simulink model "StoneVsAir"  (Simulink 7.6)
settings: Solver=ode5  StartTime=0.0  StopTime=10.0  FixedStep=0.01  RelTol=1e-3
libraries: simulink x1
settings Model: Creator=Podolsky  LastModifiedBy=Podolsky
settings DataIOCC: SignalLoggingName=sigsOut
settings DebuggingCC: SaveWithParameterizedLinksMsg=none  SignalResolutionControl=TryResolveAllWithWarning  SolverPrmCheckMsg=none  MultiTaskDSMMsg=warning  MultiTaskCondExecSysMsg=none  StrictBusMsg=None
settings HardwareCC: TargetUnknown=on
settings RTWCC: IncludeERTFirstTime=on

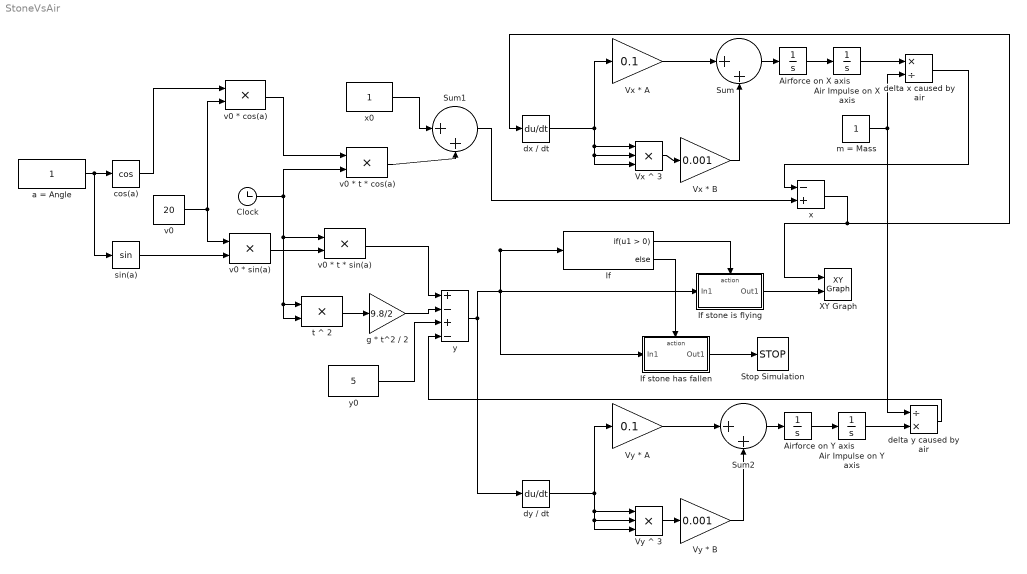
== system StoneVsAir ==
  Air Impulse on X axis : Integrator
  Air Impulse on Y axis : Integrator
  Airforce on X axis : Integrator
  Airforce on Y axis : Integrator
  Clock : Clock
      settings: Decimation=5
  If : If
  If stone has fallen : Subsystem  TreatAsAtomicUnit=on
  If stone is flying : Subsystem  TreatAsAtomicUnit=on
  Stop Simulation : Stop
  Sum : Sum  Inputs=|++
  Sum1 : Sum  Inputs=|++
  Sum2 : Sum  Inputs=|++
  Vx * A : Gain  Gain=0.1
  Vx * B : Gain  Gain=0.001
  Vx ^ 3 : Product  Inputs=3  RndMeth=Zero
  Vy * A : Gain  Gain=0.1
  Vy * B : Gain  Gain=0.001
  Vy ^ 3 : Product  Inputs=3  RndMeth=Zero
  XY Graph : simulink/Sinks/XY Graph  SystemSampleTime=-1  xmin=0  xmax=42  ymin=0  ymax=42  st=-1
  a = Angle : Constant
  cos(a) : Trigonometry  Operator=cos
  delta x caused by air : Product  Inputs=*/
  delta y caused by air : Product  Inputs=/*
  dx / dt : Derivative
  dy / dt : Derivative
  g * t^2 / 2 : Gain  Gain=9.8/2  SaturateOnIntegerOverflow=on  OutDataTypeStr=Inherit: Same as input  ParamDataTypeStr=Inherit: Same as input
  m = Mass : Constant
  sin(a) : Trigonometry
  t ^ 2 : Product  SaturateOnIntegerOverflow=on  OutDataTypeStr=Inherit: Same as first input
  v0 : Constant  Value=20
  v0 * cos(a) : Product  SaturateOnIntegerOverflow=on  OutDataTypeStr=Inherit: Same as first input
  v0 * sin(a) : Product  SaturateOnIntegerOverflow=on  OutDataTypeStr=Inherit: Same as first input
  v0 * t * cos(a) : Product  SaturateOnIntegerOverflow=on  OutDataTypeStr=Inherit: Same as first input
  v0 * t * sin(a) : Product  SaturateOnIntegerOverflow=on  OutDataTypeStr=Inherit: Same as first input
  x : Sum  Inputs=-+
  x0 : Constant
  y : Sum  Inputs=+-+-
  y0 : Constant  Value=5
  wires:
  a = Angle/1 -> cos(a)/1, sin(a)/1
  t ^ 2/1 -> g * t^2 / 2/1
  Clock/1 -> v0 * t * sin(a)/1, t ^ 2/1, t ^ 2/2, v0 * t * cos(a)/2
  y/1 -> If/1, If stone is flying/1(In1), If stone has fallen/1(In1), dy / dt/1
  If/1 -> If stone is flying/Action
  If stone is flying/1(Out1) -> XY Graph/2
  If/2 -> If stone has fallen/Action
  If stone has fallen/1(Out1) -> Stop Simulation/1
  x0/1 -> Sum1/1
  v0 * t * cos(a)/1 -> Sum1/2
  v0/1 -> v0 * cos(a)/2, v0 * sin(a)/1
  sin(a)/1 -> v0 * sin(a)/2
  cos(a)/1 -> v0 * cos(a)/1
  v0 * sin(a)/1 -> v0 * t * sin(a)/2
  v0 * cos(a)/1 -> v0 * t * cos(a)/1
  g * t^2 / 2/1 -> y/2
  v0 * t * sin(a)/1 -> y/1
  y0/1 -> y/3
  Sum1/1 -> x/2
  dx / dt/1 -> Vx * A/1, Vx ^ 3/1, Vx ^ 3/2, Vx ^ 3/3
  Vx ^ 3/1 -> Vx * B/1
  Vx * B/1 -> Sum/2
  Vx * A/1 -> Sum/1
  Sum/1 -> Airforce on X axis/1
  Airforce on X axis/1 -> Air Impulse on X axis/1
  Air Impulse on X axis/1 -> delta x caused by air/1
  m = Mass/1 -> delta x caused by air/2, delta y caused by air/1
  x/1 -> XY Graph/1, dx / dt/1
  delta x caused by air/1 -> x/1
  dy / dt/1 -> Vy ^ 3/3, Vy ^ 3/2, Vy ^ 3/1, Vy * A/1
  Vy ^ 3/1 -> Vy * B/1
  Vy * B/1 -> Sum2/2
  Vy * A/1 -> Sum2/1
  Sum2/1 -> Airforce on Y axis/1
  Airforce on Y axis/1 -> Air Impulse on Y axis/1
  Air Impulse on Y axis/1 -> delta y caused by air/2
  delta y caused by air/1 -> y/4

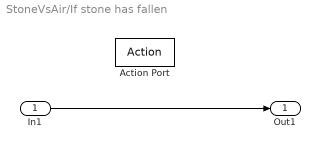
== system StoneVsAir/If stone has fallen ==
  In1 : Inport
  Action Port : ActionPort  ActionType=else
  Out1 : Outport
  wires:
  In1/1 -> Out1/1

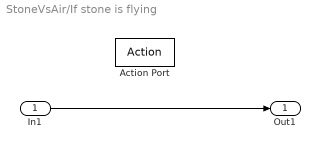
== system StoneVsAir/If stone is flying ==
  In1 : Inport
  Action Port : ActionPort  ActionType=then
  Out1 : Outport
  wires:
  In1/1 -> Out1/1
